simulink model "HydBrakeCU_ESP"  (Simulink 10.1)
settings: Solver=ode45  StartTime=0.0  StopTime=inf  RelTol=1e-3  EnableMultiTasking=on
PreLoadFcn:
  | HydBrakeCU_ESP_params
undefined symbols (not defined in the file): Area_Front, Area_Rear, ay_max_off, ay_max_on, ay_per_mu_max_off, ay_per_mu_max_on, Brake_ratio, brake_valve_ctrl_kP, cat1mode1_higher, cat1mode1_lower, cat1mode2_higher, cat1mode2_lower, cat1mode3_higher, cat1mode3_lower, cat2mode1_higher, cat2mode1_lower, cat2mode2_higher, cat2mode2_lower, cat2mode3_higher, cat2mode3_lower, delta_vel, diff_lock_fac, diff_lock_off, diff_lock_on, ESP_ctrl_kD, ESP_ctrl_kI, ESP_ctrl_kP, ESP_ctrl_restore_kI, ESP_min_throttle_fac, f_ax, f_slip, g, higherlimit_highvel, higherlimit_lowvel, highervel_fac, highervelocity_fac, InitialConditionForIntegrator, limit_acc, limit_selectlow, limit_starting, limit_vdiff, locktime_throttle, lowerlimit_highvel, lowerlimit_lowvel, lowervel_fac, lowervelocity_fac, min_throttle, MPS2KMPH, MSR_ctrl_kD, MSR_ctrl_kI, MSR_ctrl_kP, MSR_min_throttle_fac, PID_kP_sideslip, PID_kP_yawrate, RADpS2RpM, rBrake, RpM2RADpS, SH_SL_switch, sideslip_vel_corr, sidesplip_deviation_max ... (+33)
libraries: CarMaker4SL x136, simulink x49, simulink_extras x6
(part 5 of 6)

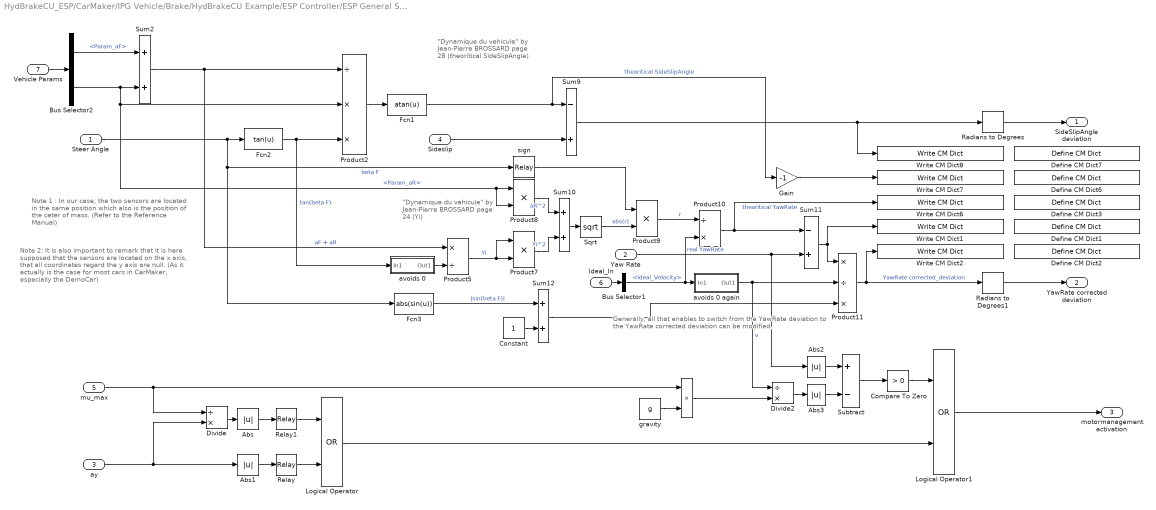
== system HydBrakeCU_ESP/CarMaker/IPG Vehicle/Brake/HydBrakeCU Example/ESP Controller/ESP General System/ESP/ECU/Instability detectors ==
  note: Note 1 :
      | In our case, the two sensors
      | are located in the same position
      | which also is the position of the ceter of mass.
      | (Refer to the Reference Manual)
  note: Note 2:
      | It is also important to remark that it is here
      | supposed that the sensors are located on the x axis,
      | that all coordinates regard the y axis are null.
      | (As it actually is the case for most cars in CarMaker,
      | especially the DemoCar)
  note: "Dynamique du vehicule"
      | by Jean-Pierre BROSSARD
      | page 28
      | (theoritical SideSlipAngle)
  note: Generally, all that enables to switch from the YawRate deviation
      | to the YawRate corrected deviation can be modified.
  note: "Dynamique du vehicule"
      | by Jean-Pierre BROSSARD
      | page 24
      | (Yi)
  Steer Angle : Inport
  Yaw Rate : Inport  Port=2
  ay : Inport  Port=3
  Sideslip : Inport  Port=4
  mu_max : Inport  Port=5
  Ideal_In : Inport  Port=6
  Vehicle Params : Inport  Port=7
  " " : Product  Inputs=**
  Abs{,1..3} (4 alike) : Abs
  Bus Selector1 : BusSelector  OutputSignals=Ideal_Velocity.Ideal_Velocity
  Bus Selector2 : BusSelector  OutputSignals=VehicleGeometry.Param_aF,VehicleGeometry.Param_aR
  Compare To Zero : simulink/Logic and Bit Operations/Compare To Zero  relop=>  OutDataTypeStr=uint8
  Constant : Constant
  Define CM Dict1 : CarMaker4SL/Define CM Dict  xname=ESP.YawRate_deviation  xunit=rad/s  xmono=off  xtype=Double4  xdvaplace=None  xnstates=0  xfirststate=0  xinitial=0
  Define CM Dict2 : CarMaker4SL/Define CM Dict  xname=ESP.YawRate_corrected_deviation  xunit=rad/m  xmono=off  xtype=Double4  xdvaplace=None  xnstates=0  xfirststate=0  xinitial=0
  Define CM Dict3 : CarMaker4SL/Define CM Dict  xname=ESP.YawRate_theoretical  xunit=rad/s  xmono=off  xtype=Double4  xdvaplace=None  xnstates=0  xfirststate=0  xinitial=0
  Define CM Dict6 : CarMaker4SL/Define CM Dict  xname=ESP.SideSlipeAngle_theoretical  xunit=rad  xmono=off  xtype=Double4  xdvaplace=None  xnstates=0  xfirststate=0  xinitial=0
  Define CM Dict7 : CarMaker4SL/Define CM Dict  xname=ESP.SideSlipAngle_deviation  xunit=rad  xmono=off  xtype=Double4  xdvaplace=None  xnstates=0  xfirststate=0  xinitial=0
  Divide : Product  Inputs=/*
  Divide2 : Product  Inputs=/*
  Fcn1 : Fcn  Expr=atan(u)
  Fcn2 : Fcn  Expr=tan(u)
  Fcn3 : Fcn  Expr=abs(sin(u))
  Gain : Gain  Gain=-1
  Logical Operator : Logic  Operator=OR  AllPortsSameDT=off  OutDataTypeStr=boolean
  Logical Operator1 : Logic  Operator=OR  AllPortsSameDT=off  OutDataTypeStr=boolean
  Product10 : Product  Inputs=/*  RndMeth=Zero
  Product11 : Product  Inputs=*/*  RndMeth=Zero
  Product2 : Product  Inputs=/**  RndMeth=Zero
  Product5 : Product  Inputs=*/  RndMeth=Zero
  Product7 : Product  RndMeth=Zero
  Product8 : Product  RndMeth=Zero
  Product9 : Product  RndMeth=Zero
  Radians to Degrees : simulink_extras/Transformations/Radians to Degrees
  Radians to Degrees1 : simulink_extras/Transformations/Radians to Degrees
  Relay : Relay  OnSwitchValue=ay_max_on  OffSwitchValue=ay_max_off
  Relay1 : Relay  OnSwitchValue=ay_per_mu_max_on  OffSwitchValue=ay_per_mu_max_off
  Sqrt : Math  Operator=sqrt  SignedPower=on  SaturateOnIntegerOverflow=on
  Subtract : Sum  Inputs=+-
  Sum10 : Sum  Inputs=2  InputSameDT=on  SaturateOnIntegerOverflow=on  OutDataTypeStr=Inherit: Same as first input
  Sum11 : Sum  Inputs=-+  InputSameDT=on  SaturateOnIntegerOverflow=on  OutDataTypeStr=Inherit: Same as first input
  Sum12 : Sum  InputSameDT=on  SaturateOnIntegerOverflow=on  OutDataTypeStr=Inherit: Same as first input
  Sum2 : Sum  Inputs=2  InputSameDT=on  SaturateOnIntegerOverflow=on  OutDataTypeStr=Inherit: Same as first input
  Sum9 : Sum  Inputs=-+  InputSameDT=on  SaturateOnIntegerOverflow=on  OutDataTypeStr=Inherit: Same as first input
  Write CM Dict1 : CarMaker4SL/Write CM Dict  xname=ESP.YawRate_deviation  xsync=off
  Write CM Dict2 : CarMaker4SL/Write CM Dict  xname=ESP.YawRate_corrected_deviation  xsync=off
  Write CM Dict6 : CarMaker4SL/Write CM Dict  xname=ESP.YawRate_theoretical  xsync=off
  Write CM Dict7 : CarMaker4SL/Write CM Dict  xname=ESP.SideSlipeAngle_theoretical  xsync=off
  Write CM Dict8 : CarMaker4SL/Write CM Dict  xname=ESP.SideSlipAngle_deviation  xsync=off
  avoids 0 : Subsystem
  avoids 0 again : Subsystem
  gravity : Constant  Value=g
  sign : Relay  OnSwitchValue=0  OffSwitchValue=0  OffOutputValue=-1
  SideSlipAngle deviation : Outport  VectorParamsAs1DForOutWhenUnconnected=off
  YawRate corrected deviation : Outport  Port=2  VectorParamsAs1DForOutWhenUnconnected=off
  motormanagement activation : Outport  Port=3  VectorParamsAs1DForOutWhenUnconnected=off
  wires:
  Steer Angle/1 -> Fcn2/1, sign/1, Fcn3/1  "beta F"
  Bus Selector2/1 -> Sum2/1  "<Param_aF>"
  Bus Selector2/2 -> Product8/1, Product8/2, Product2/2, Sum2/2  "<Param_aR>"
  Fcn2/1 -> avoids 0/1(In1), Product2/3  "tan(beta F)"
  Sum2/1 -> Product5/1, Product2/1  "aF + aR"
  Sum9/1 -> Radians to Degrees/1, Write CM Dict8/1
  Product2/1 -> Fcn1/1
  Fcn1/1 -> Sum9/1, Gain/1  "theoritical SideSlipAngle"
  Sideslip/1 -> Sum9/2
  Product5/1 -> Product7/2, Product7/1  "Yi"
  Product8/1 -> Sum10/1  "aR^2"
  Product7/1 -> Sum10/2  "Yi^2"
  Sum10/1 -> Sqrt/1
  Sqrt/1 -> Product9/2  "abs(r)"
  sign/1 -> Product9/1
  avoids 0/1(Out1) -> Product5/2
  Product9/1 -> Product10/1  "r"
  Product10/1 -> Sum11/1, Write CM Dict6/1  "theoritical YawRate"
  Yaw Rate/1 -> Sum11/2, Abs2/1  "real YawRate"
  Bus Selector1/1 -> Product10/2, avoids 0 again/1(In1)  "<Ideal_Velocity>"
  Constant/1 -> Sum12/2
  Product11/1 -> Radians to Degrees1/1, Write CM Dict2/1  "YawRate corrected_deviation"
  Sum11/1 -> Product11/1, Write CM Dict1/1
  Fcn3/1 -> Sum12/1  "|sin(beta F)|"
  avoids 0 again/1(Out1) -> Divide2/1, Product11/2  "v"
  Radians to Degrees/1 -> SideSlipAngle deviation/1
  Radians to Degrees1/1 -> YawRate corrected deviation/1
  Sum12/1 -> Product11/3
  Divide/1 -> Abs/1
  Abs/1 -> Relay1/1
  Abs1/1 -> Relay/1
  ay/1 -> Divide/2, Abs1/1
  mu_max/1 -> Divide/1, " "/1
  gravity/1 -> " "/2
  " "/1 -> Divide2/2
  Divide2/1 -> Abs3/1
  Abs2/1 -> Subtract/1
  Abs3/1 -> Subtract/2
  Subtract/1 -> Compare To Zero/1
  Logical Operator1/1 -> motormanagement activation/1
  Compare To Zero/1 -> Logical Operator1/1
  Logical Operator/1 -> Logical Operator1/2
  Relay1/1 -> Logical Operator/1
  Relay/1 -> Logical Operator/2
  Ideal_In/1 -> Bus Selector1/1
  Vehicle Params/1 -> Bus Selector2/1
  Gain/1 -> Write CM Dict7/1

== system HydBrakeCU_ESP/CarMaker/IPG Vehicle/Brake/HydBrakeCU Example/ESP Controller/ESP General System/ESP/ECU/Motor management strategy ==
  activation DK : Inport
  Throttle_position : Inport  Port=2
  ax : Inport  Port=3
  Abs1 : Abs
  Compare To Zero : simulink/Logic and Bit Operations/Compare To Zero  relop===  OutDataTypeStr=uint8
  Constant : Constant  Value=ESP_min_throttle_fac
  Data Type Conversion2 : DataTypeConversion
  PID-Controller : Subsystem
  Product : Product  RndMeth=Zero
  Saturation Dynamic : simulink/Discontinuities/Saturation Dynamic  OutMin=[]  OutMax=[]  OutDataTypeStr=Inherit: Same as second input  OutDataType=sfix(16)  OutScaling=2^-10  DoSatur=off
  Switch1 : Switch  Criteria=u2 > Threshold
  Switch3 : Switch  Criteria=u2 > Threshold
  restoration to driver : Subsystem
  vquer_VA1 : Gain
  Gas_out : Outport  VectorParamsAs1DForOutWhenUnconnected=off
  wires:
  Compare To Zero/1 -> Data Type Conversion2/1
  Data Type Conversion2/1 -> PID-Controller/2(RESET)
  Throttle_position/1 -> Switch3/3, Product/1, vquer_VA1/1
  vquer_VA1/1 -> Saturation Dynamic/1
  Product/1 -> Saturation Dynamic/3
  activation DK/1 -> Compare To Zero/1, Switch3/2, restoration to driver/2(activation on)
  PID-Controller/1(y) -> Saturation Dynamic/2
  Saturation Dynamic/1 -> Switch3/1, restoration to driver/1(controller in)
  Switch3/1 -> Switch1/3, restoration to driver/3(driver in)
  Switch1/1 -> Gas_out/1
  restoration to driver/1(Control Gas) -> Switch1/1
  ax/1 -> Abs1/1
  Abs1/1 -> PID-Controller/1(u)
  restoration to driver/2(restoration) -> Switch1/2
  Constant/1 -> Product/2

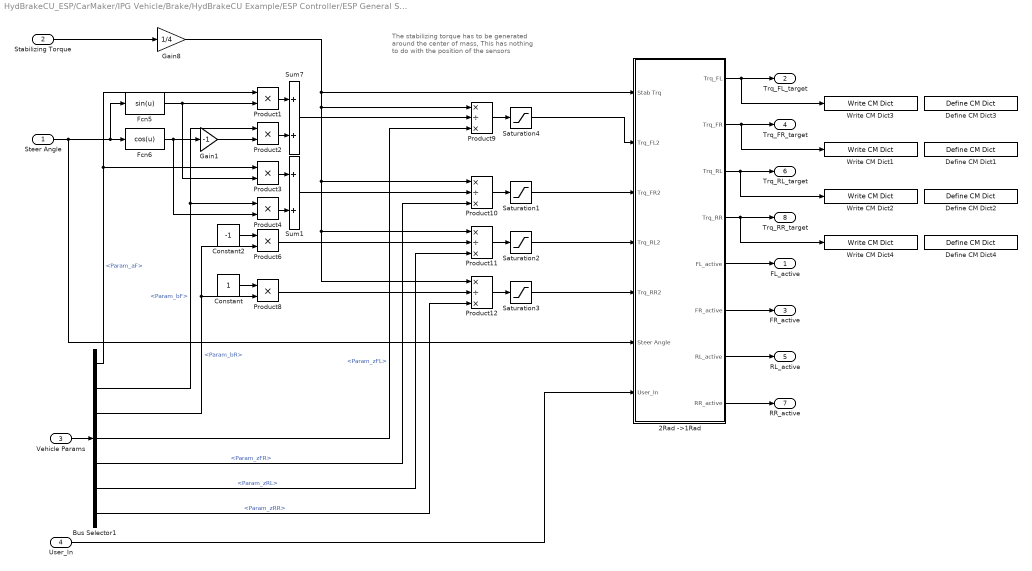
== system HydBrakeCU_ESP/CarMaker/IPG Vehicle/Brake/HydBrakeCU Example/ESP Controller/ESP General System/ESP/ECU/brake distribution strategy ==
  note: The stabilizing torque has to be generated
      | around the center of mass,
      | This has nothing to do with
      | the position of the sensors
  Steer Angle : Inport
  Stabilizing Torque : Inport  Port=2
  Vehicle Params : Inport  Port=3
  User_In : Inport  Port=4
  2Rad ->1Rad : Subsystem
  Bus Selector1 : BusSelector  OutputSignals=VehicleGeometry.Param_aF,VehicleGeometry.Param_bF,VehicleGeometry.Param_bR,CarrierGeometry.Param_zFL,CarrierGeometry.Param_zFR,CarrierGeometry.Param_zRL,CarrierGeometry.Param_zRR
  Constant : Constant
  Constant2 : Constant  Value=-1
  Define CM Dict1 : CarMaker4SL/Define CM Dict  xname=ESP.ESP_corr_Trq_FR  xunit=Nm  xmono=off  xtype=Double4  xdvaplace=None  xnstates=0  xfirststate=0  xinitial=0
  Define CM Dict2 : CarMaker4SL/Define CM Dict  xname=ESP.ESP_corr_Trq_RL  xunit=Nm  xmono=off  xtype=Double4  xdvaplace=None  xnstates=0  xfirststate=0  xinitial=0
  Define CM Dict3 : CarMaker4SL/Define CM Dict  xname=ESP.ESP_corr_Trq_FL  xunit=Nm  xmono=off  xtype=Double4  xdvaplace=None  xnstates=0  xfirststate=0  xinitial=0
  Define CM Dict4 : CarMaker4SL/Define CM Dict  xname=ESP.ESP_corr_Trq_RR  xunit=Nm  xmono=off  xtype=Double4  xdvaplace=None  xnstates=0  xfirststate=0  xinitial=0
  Fcn5 : Fcn  Expr=sin(u)
  Fcn6 : Fcn  Expr=cos(u)
  Gain1 : Gain  Gain=-1
  Gain8 : Gain  Gain=1/4
  Product{1..4,6,8} (6 alike) : Product  RndMeth=Zero
  Product{9..12} (4 alike) : Product  Inputs=*/*  RndMeth=Zero
  Saturation{1..4} (4 alike) : Saturate  UpperLimit=3000  LowerLimit=-3000
  Sum1 : Sum  Inputs=2  InputSameDT=on  SaturateOnIntegerOverflow=on  OutDataTypeStr=Inherit: Same as first input
  Sum7 : Sum  Inputs=2  InputSameDT=on  SaturateOnIntegerOverflow=on  OutDataTypeStr=Inherit: Same as first input
  Write CM Dict1 : CarMaker4SL/Write CM Dict  xname=ESP.ESP_corr_Trq_FR  xsync=off
  Write CM Dict2 : CarMaker4SL/Write CM Dict  xname=ESP.ESP_corr_Trq_RL  xsync=off
  Write CM Dict3 : CarMaker4SL/Write CM Dict  xname=ESP.ESP_corr_Trq_FL  xsync=off
  Write CM Dict4 : CarMaker4SL/Write CM Dict  xname=ESP.ESP_corr_Trq_RR  xsync=off
  FL_active : Outport  VectorParamsAs1DForOutWhenUnconnected=off
  Trq_FL_target : Outport  Port=2  VectorParamsAs1DForOutWhenUnconnected=off
  FR_active : Outport  Port=3  VectorParamsAs1DForOutWhenUnconnected=off
  Trq_FR_target : Outport  Port=4  VectorParamsAs1DForOutWhenUnconnected=off
  RL_active : Outport  Port=5  VectorParamsAs1DForOutWhenUnconnected=off
  Trq_RL_target : Outport  Port=6  VectorParamsAs1DForOutWhenUnconnected=off
  RR_active : Outport  Port=7  VectorParamsAs1DForOutWhenUnconnected=off
  Trq_RR_target : Outport  Port=8  VectorParamsAs1DForOutWhenUnconnected=off
  wires:
  Steer Angle/1 -> Fcn5/1, Fcn6/1, 2Rad ->1Rad/6(Steer Angle)
  Fcn5/1 -> Product1/2, Product3/2
  Fcn6/1 -> Product4/2, Gain1/1
  Gain1/1 -> Product2/2
  Product1/1 -> Sum7/1
  Product2/1 -> Sum7/2
  Product3/1 -> Sum1/1
  Product4/1 -> Sum1/2
  Product6/1 -> Product11/2
  Product8/1 -> Product12/2
  Sum1/1 -> Product10/2
  Sum7/1 -> Product9/2
  Product9/1 -> Saturation4/1
  Saturation4/1 -> 2Rad ->1Rad/2(Trq_FL2)
  Saturation1/1 -> 2Rad ->1Rad/3(Trq_FR2)
  Saturation3/1 -> 2Rad ->1Rad/5(Trq_RR2)
  Saturation2/1 -> 2Rad ->1Rad/4(Trq_RL2)
  Stabilizing Torque/1 -> Gain8/1
  Gain8/1 -> Product12/1, Product11/1, Product10/1, Product9/1, 2Rad ->1Rad/1(Stab Trq)
  Product10/1 -> Saturation1/1
  Product12/1 -> Saturation3/1
  Product11/1 -> Saturation2/1
  Bus Selector1/3 -> Product6/2, Product8/2  "<Param_bR>"
  Bus Selector1/2 -> Product4/1, Product2/1  "<Param_bF>"
  2Rad ->1Rad/2(Trq_FR) -> Write CM Dict1/1, Trq_FR_target/1
  2Rad ->1Rad/3(Trq_RL) -> Write CM Dict2/1, Trq_RL_target/1
  2Rad ->1Rad/4(Trq_RR) -> Trq_RR_target/1, Write CM Dict4/1
  2Rad ->1Rad/5(FL_active) -> FL_active/1
  2Rad ->1Rad/6(FR_active) -> FR_active/1
  2Rad ->1Rad/7(RL_active) -> RL_active/1
  2Rad ->1Rad/8(RR_active) -> RR_active/1
  Vehicle Params/1 -> Bus Selector1/1
  Bus Selector1/1 -> Product3/1, Product1/1  "<Param_aF>"
  Constant2/1 -> Product6/1
  Constant/1 -> Product8/1
  Bus Selector1/4 -> Product9/3  "<Param_zFL>"
  Bus Selector1/5 -> Product10/3  "<Param_zFR>"
  Bus Selector1/6 -> Product11/3  "<Param_zRL>"
  Bus Selector1/7 -> Product12/3  "<Param_zRR>"
  User_In/1 -> 2Rad ->1Rad/7(User_In)
  2Rad ->1Rad/1(Trq_FL) -> Write CM Dict3/1, Trq_FL_target/1

== system HydBrakeCU_ESP/CarMaker/IPG Vehicle/Brake/HydBrakeCU Example/ESP Controller/ESP General System/ESP/helpsignals estimator/SideSlip estimator ==
  lenkwinkel : Inport
  CarMaker_In : Inport  Port=2
  Bus Selector1 : BusSelector  OutputSignals=Ideal_Velocity.Ideal_Velocity_y,Ideal_Velocity.Ideal_Velocity_x
  Constant1 : Constant  Value=0
  Divide6 : Product  Inputs=*/
  Switch : Switch  Threshold=1
  Terminator : Terminator
  Trigonometric Function2 : Trigonometry  Operator=atan
  SideSlipAngle_estimated : Outport  VectorParamsAs1DForOutWhenUnconnected=off
  wires:
  Bus Selector1/2 -> Divide6/2, Switch/2  "<Ideal_Velocity_x>"
  Divide6/1 -> Trigonometric Function2/1
  Trigonometric Function2/1 -> Switch/1
  Constant1/1 -> Switch/3
  Switch/1 -> SideSlipAngle_estimated/1
  lenkwinkel/1 -> Terminator/1
  CarMaker_In/1 -> Bus Selector1/1
  Bus Selector1/1 -> Divide6/1  "<Ideal_Velocity_y>"

== system HydBrakeCU_ESP/CarMaker/IPG Vehicle/Brake/HydBrakeCU Example/ESP Controller/ESP General System/ESP/helpsignals estimator/mue estimator ==
  CarMaker_In : Inport
  Vehicle Params : Inport  Port=2
  Bus Selector1 : BusSelector  OutputSignals=Idea_Trq2W.Ideal_Trq2WRL,Ideal_Fz.Ideal_FzRL,Ideal_Slip.Ideal_SlipRL,Ideal_Velocity.Ideal_Velocity_x,Ideal_YawRate
  Bus Selector2 : BusSelector  OutputSignals=TireRadius.Param_RadiusRL,TireRadius.Param_RadiusRR
  Bus Selector3 : BusSelector  OutputSignals=Idea_Trq2W.Ideal_Trq2WRR,Ideal_Fz.Ideal_FzRR,Ideal_Slip.Ideal_SlipRR,Ideal_Velocity.Ideal_Velocity_x,Ideal_YawRate
  MinMax : MinMax  Inputs=2
  estimator_RL : Subsystem
  estimator_RR : Subsystem
  mue_estimated : Outport  VectorParamsAs1DForOutWhenUnconnected=off
  wires:
  MinMax/1 -> mue_estimated/1
  estimator_RL/1(mue_est_RL) -> MinMax/1
  estimator_RR/1(mue_est_RR) -> MinMax/2
  CarMaker_In/1 -> Bus Selector3/1, Bus Selector1/1
  Vehicle Params/1 -> Bus Selector2/1
  Bus Selector2/1 -> estimator_RL/6(Radius_RL)  "<Param_RadiusRL>"
  Bus Selector2/2 -> estimator_RR/6(Radius_RR)  "<Param_RadiusRR>"
  Bus Selector1/3 -> estimator_RL/3(LongSlip_RL)  "<Ideal_SlipRL>"
  Bus Selector1/4 -> estimator_RL/4(Car_vx)  "<Ideal_Velocity_x>"
  Bus Selector1/2 -> estimator_RL/2(Fz_RL)  "<Ideal_FzRL>"
  Bus Selector1/5 -> estimator_RL/5(YawRate)  "<Ideal_YawRate>"
  Bus Selector1/1 -> estimator_RL/1(Trq2W_RL)  "<Ideal_Trq2WRL>"
  Bus Selector3/1 -> estimator_RR/1(Trq2W_RR)  "<Ideal_Trq2WRR>"
  Bus Selector3/2 -> estimator_RR/2(Fz_RR)  "<Ideal_FzRR>"
  Bus Selector3/3 -> estimator_RR/3(LongSlip_RR)  "<Ideal_SlipRR>"
  Bus Selector3/4 -> estimator_RR/4(Car_vx)  "<Ideal_Velocity_x>"
  Bus Selector3/5 -> estimator_RR/5(YawRate)  "<Ideal_YawRate>"

== system HydBrakeCU_ESP/CarMaker/IPG Vehicle/Brake/HydBrakeCU Example/ESP Controller/ESP General System/ABS/ABS ECU/ABS_ValveCtrl_FL/Duty ==
  Constant1 : Constant  Value=1/t_Sensor
  Integrator : Integrator  ExternalReset=either
  Pulse Generator : DiscretePulseGenerator  PulseType=Time based  Period=t_Sensor*2  PulseWidth=50
  SZ : Outport  VectorParamsAs1DForOutWhenUnconnected=off
  wires:
  Pulse Generator/1 -> Integrator/2
  Constant1/1 -> Integrator/1
  Integrator/1 -> SZ/1

== system HydBrakeCU_ESP/CarMaker/IPG Vehicle/Brake/HydBrakeCU Example/ESP Controller/ESP General System/ABS/ABS ECU/ABS_ValveCtrl_FR/Duty ==
  Constant1 : Constant  Value=1/t_Sensor
  Integrator : Integrator  ExternalReset=either
  Pulse Generator : DiscretePulseGenerator  PulseType=Time based  Period=t_Sensor*2  PulseWidth=50
  SZ : Outport  VectorParamsAs1DForOutWhenUnconnected=off
  wires:
  Integrator/1 -> SZ/1
  Pulse Generator/1 -> Integrator/2
  Constant1/1 -> Integrator/1

== system HydBrakeCU_ESP/CarMaker/IPG Vehicle/Brake/HydBrakeCU Example/ESP Controller/ESP General System/ABS/ABS ECU/select_low/ABS_ValveCtrl_rear ==
  note: Valve Control:
      | Valves are open for a predefined time window.
      | The driving time depends on a trigger criterion (LUT).
      | The treshold change for the valve driving time is
      | continously modified by a repeating sequence.
  note: EITHER ABS is switched on and  S_K is put through
      |  when S_K is becomming bigger the s_{ku}
      | OR output is 0 when S_K is smaller than {sku}_{off}
  Sk : Inport
  Constant : Constant
  Duty : Subsystem
  Look-Up Table1 : Lookup  InputValues=Valve_LUTin_HA  Table=ValveIn_LUTout_HA  LookUpMeth=Interpolation-Use End Values  SaturateOnIntegerOverflow=on
  Look-Up Table2 : Lookup  InputValues=Valve_LUTin_HA  Table=ValveOut_LUTout_HA  LookUpMeth=Interpolation-Use End Values  SaturateOnIntegerOverflow=on
  Product : Product  SaturateOnIntegerOverflow=on  OutDataTypeStr=Inherit: Same as first input
  Rate Transition{1..4} (4 alike) : RateTransition
  Relational Operator : RelationalOperator  Operator=<  SampleTime=0.001  RndMeth=Nearest
  Relational Operator1 : RelationalOperator  Operator=<  SampleTime=0.001  RndMeth=Nearest
  Relay : Relay  OnSwitchValue=sku_HA  OffSwitchValue=sku_off_HA
  Sum1 : Sum  Inputs=--+  SaturateOnIntegerOverflow=on
  Zero-Order Hold : ZeroOrderHold  SampleTime=t_Sensor
  Brake.Valve.In : Outport  VectorParamsAs1DForOutWhenUnconnected=off
  Brake.Valve.Out : Outport  Port=2  VectorParamsAs1DForOutWhenUnconnected=off
  Brake.ABS.status : Outport  Port=3  VectorParamsAs1DForOutWhenUnconnected=off
  Brake.ABS.on/off : Outport  Port=4  VectorParamsAs1DForOutWhenUnconnected=off
  wires:
  Sk/1 -> Zero-Order Hold/1
  Product/1 -> Look-Up Table1/1, Look-Up Table2/1
  Relay/1 -> Rate Transition4/1, Product/2
  Zero-Order Hold/1 -> Product/1, Relay/1
  Look-Up Table2/1 -> Rate Transition3/1
  Look-Up Table1/1 -> Rate Transition1/1
  Duty/1(SZ) -> Rate Transition2/1
  Sum1/1 -> Brake.ABS.status/1
  Constant/1 -> Sum1/3
  Relational Operator1/1 -> Sum1/2, Brake.Valve.Out/1
  Relational Operator/1 -> Sum1/1, Brake.Valve.In/1
  Rate Transition2/1 -> Relational Operator1/1, Relational Operator/1
  Rate Transition1/1 -> Relational Operator/2
  Rate Transition3/1 -> Relational Operator1/2
  Rate Transition4/1 -> Brake.ABS.on/off/1

== system HydBrakeCU_ESP/CarMaker/IPG Vehicle/Brake/HydBrakeCU Example/ESP Controller/ESP General System/ASR/BMR ECU/BMR Controller/If Action Subsystem10 ==
  Action Port : ActionPort  ActionPortLabel=else { }
  Constant3 : Constant  Value=ValveIn_abbau
  Constant4 : Constant  Value=ValveOut_abbau
  Out1 : Outport  InitialOutput=[ValveIn_abbau]  VectorParamsAs1DForOutWhenUnconnected=off
  Out2 : Outport  Port=2  InitialOutput=[ValveOut_abbau]  VectorParamsAs1DForOutWhenUnconnected=off
  wires:
  Constant3/1 -> Out1/1
  Constant4/1 -> Out2/1

== system HydBrakeCU_ESP/CarMaker/IPG Vehicle/Brake/HydBrakeCU Example/ESP Controller/ESP General System/ASR/BMR ECU/BMR Controller/If Action Subsystem11 ==
  Action Port : ActionPort  ActionPortLabel=else { }
  Constant3 : Constant  Value=ValveIn_abbau
  Constant4 : Constant  Value=ValveOut_abbau
  Out1 : Outport  InitialOutput=[ValveIn_abbau]  VectorParamsAs1DForOutWhenUnconnected=off
  Out2 : Outport  Port=2  InitialOutput=[ValveOut_abbau]  VectorParamsAs1DForOutWhenUnconnected=off
  wires:
  Constant3/1 -> Out1/1
  Constant4/1 -> Out2/1

== system HydBrakeCU_ESP/CarMaker/IPG Vehicle/Brake/HydBrakeCU Example/ESP Controller/ESP General System/ASR/BMR ECU/BMR Controller/If Action Subsystem12 ==
  Action Port : ActionPort  ActionPortLabel=if { }
  Constant2 : Constant  Value=ValveIn_aufbau_long
  Constant3 : Constant  Value=ValveOut_aufbau_long
  Out1 : Outport  InitialOutput=[ValveIn_aufbau_long]  VectorParamsAs1DForOutWhenUnconnected=off
  Out2 : Outport  Port=2  InitialOutput=[ValveOut_aufbau_long]  VectorParamsAs1DForOutWhenUnconnected=off
  wires:
  Constant3/1 -> Out2/1
  Constant2/1 -> Out1/1

== system HydBrakeCU_ESP/CarMaker/IPG Vehicle/Brake/HydBrakeCU Example/ESP Controller/ESP General System/ASR/BMR ECU/BMR Controller/If Action Subsystem13 ==
  Action Port : ActionPort  ActionPortLabel=elseif { }
  Constant2 : Constant  Value=ValveIn_aufbau_short
  Constant3 : Constant  Value=ValveOut_aufbau_short
  Out1 : Outport  InitialOutput=[ValveIn_aufbau_short]  VectorParamsAs1DForOutWhenUnconnected=off
  Out2 : Outport  Port=2  InitialOutput=[ValveOut_aufbau_short]  VectorParamsAs1DForOutWhenUnconnected=off
  wires:
  Constant2/1 -> Out1/1
  Constant3/1 -> Out2/1

== system HydBrakeCU_ESP/CarMaker/IPG Vehicle/Brake/HydBrakeCU Example/ESP Controller/ESP General System/ASR/BMR ECU/BMR Controller/If Action Subsystem8 ==
  Action Port : ActionPort  ActionPortLabel=if { }
  Constant2 : Constant  Value=ValveIn_aufbau_long
  Constant3 : Constant  Value=ValveOut_aufbau_long
  Out1 : Outport  InitialOutput=[ValveIn_aufbau_long]  VectorParamsAs1DForOutWhenUnconnected=off
  Out2 : Outport  Port=2  InitialOutput=[ValveOut_aufbau_long]  VectorParamsAs1DForOutWhenUnconnected=off
  wires:
  Constant2/1 -> Out1/1
  Constant3/1 -> Out2/1

== system HydBrakeCU_ESP/CarMaker/IPG Vehicle/Brake/HydBrakeCU Example/ESP Controller/ESP General System/ASR/BMR ECU/BMR Controller/If Action Subsystem9 ==
  Action Port : ActionPort  ActionPortLabel=elseif { }
  Constant2 : Constant  Value=ValveIn_aufbau_short
  Constant3 : Constant  Value=ValveOut_aufbau_short
  Out1 : Outport  InitialOutput=[ValveIn_aufbau_short]  VectorParamsAs1DForOutWhenUnconnected=off
  Out2 : Outport  Port=2  InitialOutput=[ValveOut_aufbau_short]  VectorParamsAs1DForOutWhenUnconnected=off
  wires:
  Constant2/1 -> Out1/1
  Constant3/1 -> Out2/1

== system HydBrakeCU_ESP/CarMaker/IPG Vehicle/Brake/HydBrakeCU Example/ESP Controller/ESP General System/ASR/BMR ECU/BMR Controller/Pulsing ==
  Constant1 : Constant  Value=1/t_Sensor
  Integrator : Integrator  ExternalReset=either
  Pulse Generator : DiscretePulseGenerator  PulseType=Time based  Period=t_Sensor*2  PulseWidth=50
  SZ : Outport  VectorParamsAs1DForOutWhenUnconnected=off
  wires:
  Pulse Generator/1 -> Integrator/2
  Constant1/1 -> Integrator/1
  Integrator/1 -> SZ/1

== system HydBrakeCU_ESP/CarMaker/IPG Vehicle/Brake/HydBrakeCU Example/ESP Controller/ESP General System/ASR/BMR ECU/BMR Controller/Pulsing1 ==
  Constant1 : Constant  Value=1/t_Sensor
  Integrator : Integrator  ExternalReset=either
  Pulse Generator : DiscretePulseGenerator  PulseType=Time based  Period=t_Sensor*2  PulseWidth=50
  SZ : Outport  VectorParamsAs1DForOutWhenUnconnected=off
  wires:
  Integrator/1 -> SZ/1
  Constant1/1 -> Integrator/1
  Pulse Generator/1 -> Integrator/2

== system HydBrakeCU_ESP/CarMaker/IPG Vehicle/Brake/HydBrakeCU Example/ESP Controller/ESP General System/ASR/BMR ECU/BMR Controller/Signal Mapping ==
  User_In : Inport
  Valve_In_DrivenL : Inport  Port=2
  Valve_Out_DrivenL : Inport  Port=3
  Valve_In_DrivenR : Inport  Port=4
  Valve_Out_DrivenR : Inport  Port=5
  Valve_In_Undriven : Inport  Port=6
  Valve_Out_Undriven : Inport  Port=7
  Valves_Drivenaxle : Inport  Port=8
  Valves_Undrivenaxle : Inport  Port=9
  Bus Selector2 : BusSelector  OutputSignals=User_Drive
  Demux2 : Demux  Outputs=13
  Mux1 : Mux  Inputs=13
  Mux2 : Mux  Inputs=13
  Mux3 : Mux  Inputs=13
  Switch2 : Switch  Criteria=u2 > Threshold  Threshold=1.5
  Switch3 : Switch  Criteria=u2 > Threshold  Threshold=2.5
  Brake Valve_In_FL : Outport  VectorParamsAs1DForOutWhenUnconnected=off
  Brake Valve_In_FR : Outport  Port=2  VectorParamsAs1DForOutWhenUnconnected=off
  Brake Valve_In_RL : Outport  Port=3  VectorParamsAs1DForOutWhenUnconnected=off
  Brake Valve_In_RR : Outport  Port=4  VectorParamsAs1DForOutWhenUnconnected=off
  Brake Valve_Out_FL : Outport  Port=5  VectorParamsAs1DForOutWhenUnconnected=off
  Brake Valve_Out_FR : Outport  Port=6  VectorParamsAs1DForOutWhenUnconnected=off
  Brake Valve_Out_RL : Outport  Port=7  VectorParamsAs1DForOutWhenUnconnected=off
  Brake Valve_Out_RR : Outport  Port=8  VectorParamsAs1DForOutWhenUnconnected=off
  Valve_PV_0 : Outport  Port=9  VectorParamsAs1DForOutWhenUnconnected=off
  Valve_PV_1 : Outport  Port=10  VectorParamsAs1DForOutWhenUnconnected=off
  Valve_SV_0 : Outport  Port=11  VectorParamsAs1DForOutWhenUnconnected=off
  Valve_SV_1 : Outport  Port=12  VectorParamsAs1DForOutWhenUnconnected=off
  Pump Ctrl : Outport  Port=13  VectorParamsAs1DForOutWhenUnconnected=off
  wires:
  Valve_In_Undriven/1 -> Mux2/1, Mux2/2, Mux1/5, Mux1/6
  Valve_Out_Undriven/1 -> Mux2/3, Mux2/4, Mux1/7, Mux1/8
  Valve_In_DrivenR/1 -> Mux2/7, Mux1/3, Mux3/7, Mux3/3
  Valve_In_DrivenL/1 -> Mux3/5, Mux3/1, Mux2/5, Mux1/1
  Valves_Undrivenaxle/1 -> Mux1/12, Mux1/11, Mux2/9, Mux2/10
  Valves_Drivenaxle/1 -> Mux1/9, Mux2/11, Mux2/12, Mux2/13, Mux1/10, Mux1/13, Mux3/10, Mux3/9, Mux3/11, Mux3/12, Mux3/13
  Valve_Out_DrivenL/1 -> Mux3/6, Mux3/2, Mux1/2, Mux2/6
  Valve_Out_DrivenR/1 -> Mux2/8, Mux3/4, Mux3/8, Mux1/4
  User_In/1 -> Bus Selector2/1
  Bus Selector2/1 -> Switch2/2, Switch3/2  "<User_Drive>"
  Switch2/1 -> Switch3/3
  Switch3/1 -> Demux2/1
  Mux1/1 -> Switch2/3
  Mux2/1 -> Switch2/1
  Demux2/1 -> Brake Valve_In_FL/1
  Demux2/2 -> Brake Valve_Out_FL/1
  Demux2/3 -> Brake Valve_In_FR/1
  Demux2/4 -> Brake Valve_Out_FR/1
  Demux2/5 -> Brake Valve_In_RL/1
  Demux2/6 -> Brake Valve_In_RR/1
  Demux2/7 -> Brake Valve_Out_RL/1
  Demux2/8 -> Brake Valve_Out_RR/1
  Demux2/9 -> Valve_PV_0/1
  Demux2/10 -> Valve_SV_0/1
  Demux2/11 -> Valve_PV_1/1
  Demux2/12 -> Valve_SV_1/1
  Demux2/13 -> Pump Ctrl/1
  Mux3/1 -> Switch3/1

== system HydBrakeCU_ESP/CarMaker/IPG Vehicle/Brake/HydBrakeCU Example/ESP Controller/ESP General System/ASR/BMR ECU/BMR logic/If Action Subsystem6 ==
  Action Port : ActionPort  ActionPortLabel=case: { }
  Constant : Constant  Value=higherlimit_lowvel
  Constant1 : Constant  Value=lowerlimit_lowvel
  Mux1 : Mux  Inputs=2
  1 : Outport  InitialOutput=[higherlimit_lowvel, lowerlimit_lowvel]  VectorParamsAs1DForOutWhenUnconnected=off
  wires:
  Mux1/1 -> 1/1
  Constant1/1 -> Mux1/2
  Constant/1 -> Mux1/1

== system HydBrakeCU_ESP/CarMaker/IPG Vehicle/Brake/HydBrakeCU Example/ESP Controller/ESP General System/ASR/BMR ECU/BMR logic/If Action Subsystem7 ==
  Action Port : ActionPort  ActionPortLabel=case: { }
  Constant : Constant  Value=higherlimit_highvel
  Constant1 : Constant  Value=lowerlimit_highvel
  Mux1 : Mux  Inputs=2
  2 : Outport  InitialOutput=[higherlimit_highvel, lowerlimit_highvel]  VectorParamsAs1DForOutWhenUnconnected=off
  wires:
  Constant/1 -> Mux1/1
  Constant1/1 -> Mux1/2
  Mux1/1 -> 2/1

== system HydBrakeCU_ESP/CarMaker/IPG Vehicle/Brake/HydBrakeCU Example/ESP Controller/ESP General System/ASR/BMR ECU/BMR logic/operating category ==
  note: Criteria of operating categories (Betriebsarten): Burckhardt: Fahrwerktechnik p.186f.
  v_RL : Inport
  v_RR : Inport  Port=2
  " " : RelationalOperator  Operator=>  OutDataTypeStr=boolean  RndMeth=Nearest
  "  " : Gain  Gain=0.5
  " 1" : RelationalOperator  Operator=<=  OutDataTypeStr=boolean  RndMeth=Nearest
  Add : Sum
  Add1 : Sum
  Constant1 : Constant  Value=delta_vel
  Constant2 : Constant  Value=delta_vel
  Data Type Conversion : DataTypeConversion
  Data Type Conversion1 : DataTypeConversion
  Data Type Conversion2 : DataTypeConversion
  vquer_HA2 : Gain
  vquer_HA3 : Gain  Gain=2
  operating category : Outport  VectorParamsAs1DForOutWhenUnconnected=off
  wires:
  " 1"/1 -> Data Type Conversion1/1
  " "/1 -> Data Type Conversion2/1
  Data Type Conversion/1 -> operating category/1
  Add1/1 -> Data Type Conversion/1
  vquer_HA3/1 -> Add1/2
  vquer_HA2/1 -> Add1/1
  "  "/1 -> " 1"/1, " "/1
  v_RL/1 -> Add/1
  Add/1 -> "  "/1
  v_RR/1 -> Add/2
  Constant2/1 -> " "/2
  Constant1/1 -> " 1"/2
  Data Type Conversion1/1 -> vquer_HA2/1
  Data Type Conversion2/1 -> vquer_HA3/1

== system HydBrakeCU_ESP/CarMaker/IPG Vehicle/Brake/HydBrakeCU Example/ESP Controller/ESP General System/ASR/MSR ECU/MSR logic/If Action Subsystem ==
  Action Port : ActionPort  ActionPortLabel=case: { }
  Constant : Constant  Value=cat1mode1_higher
  Constant1 : Constant  Value=cat1mode1_lower
  Mux1 : Mux  Inputs=2
  1.1 : Outport  InitialOutput=[cat1mode1_higher, cat1mode1_lower]  VectorParamsAs1DForOutWhenUnconnected=off
  wires:
  Constant/1 -> Mux1/1
  Constant1/1 -> Mux1/2
  Mux1/1 -> 1.1/1

== system HydBrakeCU_ESP/CarMaker/IPG Vehicle/Brake/HydBrakeCU Example/ESP Controller/ESP General System/ASR/MSR ECU/MSR logic/If Action Subsystem1 ==
  Action Port : ActionPort  ActionPortLabel=case: { }
  Constant : Constant  Value=cat1mode2_higher
  Constant1 : Constant  Value=cat1mode2_lower
  Mux1 : Mux  Inputs=2
  1.2 : Outport  InitialOutput=[cat1mode2_higher, cat1mode2_lower]  VectorParamsAs1DForOutWhenUnconnected=off
  wires:
  Mux1/1 -> 1.2/1
  Constant1/1 -> Mux1/2
  Constant/1 -> Mux1/1

== system HydBrakeCU_ESP/CarMaker/IPG Vehicle/Brake/HydBrakeCU Example/ESP Controller/ESP General System/ASR/MSR ECU/MSR logic/If Action Subsystem2 ==
  Action Port : ActionPort  ActionPortLabel=case: { }
  Constant2 : Constant  Value=cat1mode3_higher
  Constant3 : Constant  Value=cat1mode3_lower
  Mux1 : Mux  Inputs=2
  1.3 : Outport  InitialOutput=[cat1mode3_higher, cat1mode3_lower]  VectorParamsAs1DForOutWhenUnconnected=off
  wires:
  Mux1/1 -> 1.3/1
  Constant2/1 -> Mux1/1
  Constant3/1 -> Mux1/2

== system HydBrakeCU_ESP/CarMaker/IPG Vehicle/Brake/HydBrakeCU Example/ESP Controller/ESP General System/ASR/MSR ECU/MSR logic/If Action Subsystem3 ==
  Action Port : ActionPort  ActionPortLabel=case: { }
  Constant2 : Constant  Value=cat2mode1_higher
  Constant3 : Constant  Value=cat2mode1_lower
  Mux1 : Mux  Inputs=2
  2.1 : Outport  InitialOutput=[cat2mode1_higher, cat2mode1_lower]  VectorParamsAs1DForOutWhenUnconnected=off
  wires:
  Mux1/1 -> 2.1/1
  Constant3/1 -> Mux1/2
  Constant2/1 -> Mux1/1

== system HydBrakeCU_ESP/CarMaker/IPG Vehicle/Brake/HydBrakeCU Example/ESP Controller/ESP General System/ASR/MSR ECU/MSR logic/If Action Subsystem4 ==
  Action Port : ActionPort  ActionPortLabel=case: { }
  Constant2 : Constant  Value=cat2mode2_higher
  Constant3 : Constant  Value=cat2mode2_lower
  Mux1 : Mux  Inputs=2
  2.2 : Outport  InitialOutput=[cat2mode2_higher, cat2mode2_lower]  VectorParamsAs1DForOutWhenUnconnected=off
  wires:
  Mux1/1 -> 2.2/1
  Constant2/1 -> Mux1/1
  Constant3/1 -> Mux1/2

== system HydBrakeCU_ESP/CarMaker/IPG Vehicle/Brake/HydBrakeCU Example/ESP Controller/ESP General System/ASR/MSR ECU/MSR logic/If Action Subsystem5 ==
  Action Port : ActionPort  ActionPortLabel=case: { }
  Constant2 : Constant  Value=cat2mode3_higher
  Constant3 : Constant  Value=cat2mode3_lower
  Mux1 : Mux  Inputs=2
  2.3 : Outport  InitialOutput=[cat2mode3_higher, cat2mode3_lower]  VectorParamsAs1DForOutWhenUnconnected=off
  wires:
  Mux1/1 -> 2.3/1
  Constant2/1 -> Mux1/1
  Constant3/1 -> Mux1/2

== system HydBrakeCU_ESP/CarMaker/IPG Vehicle/Brake/HydBrakeCU Example/ESP Controller/ESP General System/ASR/MSR ECU/MSR logic/operating category ==
  note: Criteria of operating categories (Betriebsarten) - Burckhardt: Fahrwerktechnik p.174f.
  v_drivenL : Inport
  v_drivenR : Inport  Port=2
  v_undrivenL : Inport  Port=3
  v_undrivenR : Inport  Port=4
  " " : RelationalOperator  OutDataTypeStr=boolean  RndMeth=Nearest
  " 1" : RelationalOperator  Operator=<=  OutDataTypeStr=boolean  RndMeth=Nearest
  " 2" : RelationalOperator  Operator=>  OutDataTypeStr=boolean  RndMeth=Nearest
  " 3" : RelationalOperator  Operator=<  OutDataTypeStr=boolean  RndMeth=Nearest
  Abs : Abs
  Add : Sum
  Add1 : Sum
  Constant1 : Constant  Value=limit_selectlow
  Constant2 : Constant  Value=SH_SL_switch
  Constant3 : Constant  Value=SH_SL_switch
  Data Type Conversion : DataTypeConversion
  Data Type Conversion1 : DataTypeConversion
  Data Type Conversion2 : DataTypeConversion
  Logical Operator : Logic  AllPortsSameDT=off  OutDataTypeStr=boolean
  Logical Operator1 : Logic  Operator=OR  AllPortsSameDT=off  OutDataTypeStr=boolean
  Subtract : Sum  Inputs=+-
  Subtract1 : Sum  Inputs=+-
  Subtract2 : Sum  Inputs=+-
  vquer_HA : Gain  Gain=0.5
  vquer_HA2 : Gain  Gain=10
  vquer_HA3 : Gain  Gain=20
  category : Outport  VectorParamsAs1DForOutWhenUnconnected=off
  wires:
  v_undrivenR/1 -> Add/2, Subtract1/2
  Add/1 -> vquer_HA/1
  v_undrivenL/1 -> Add/1, Subtract/2
  vquer_HA/1 -> " 2"/1, " 1"/1
  vquer_HA2/1 -> Add1/1
  vquer_HA3/1 -> Add1/2
  Add1/1 -> Data Type Conversion/1
  Data Type Conversion/1 -> category/1
  Logical Operator1/1 -> Data Type Conversion2/1
  " 1"/1 -> Logical Operator/2
  Logical Operator/1 -> Data Type Conversion1/1
  v_drivenL/1 -> Subtract/1
  v_drivenR/1 -> Subtract1/1
  Subtract1/1 -> Subtract2/1
  Subtract/1 -> Subtract2/2
  Subtract2/1 -> Abs/1
  " "/1 -> Logical Operator/1
  " 3"/1 -> Logical Operator1/2
  Abs/1 -> " 3"/1, " "/1
  Constant2/1 -> " "/2
  Constant1/1 -> " 2"/2, " 1"/2
  " 2"/1 -> Logical Operator1/1
  Constant3/1 -> " 3"/2
  Data Type Conversion1/1 -> vquer_HA2/1
  Data Type Conversion2/1 -> vquer_HA3/1

== system HydBrakeCU_ESP/CarMaker/IPG Vehicle/Brake/HydBrakeCU Example/ESP Controller/ESP General System/ASR/MSR ECU/MSR logic/operating mode ==
  note: Criteria of modes (Arbeitsbereiche) - Burckhardt: Fahrwerktechnik p.174f.
  v_undrivenL : Inport
  v_undrivenR : Inport  Port=2
  " " : RelationalOperator  OutDataTypeStr=boolean  RndMeth=Nearest
  " 1" : RelationalOperator  Operator=<=  OutDataTypeStr=boolean  RndMeth=Nearest
  " 2" : RelationalOperator  Operator=>  OutDataTypeStr=boolean  RndMeth=Nearest
  " 3" : RelationalOperator  Operator=<=  OutDataTypeStr=boolean  RndMeth=Nearest
  AB1 = inaktiv : simulink/Logic and Bit Operations/Compare To Constant  relop=<  const=1  OutDataTypeStr=uint8
  AB1 = inaktiv1 : simulink/Logic and Bit Operations/Compare To Constant  relop=<  const=1  OutDataTypeStr=uint8
  Abs : Abs
  Add : Sum
  Add1 : Sum  Inputs=+++
  Constant1 : Constant  Value=limit_starting
  Constant2 : Constant  Value=limit_acc
  Constant3 : Constant  Value=limit_vdiff
  Constant4 : Constant  Value=MPS2KMPH
  Data Type Conversion{,1..3} (4 alike) : DataTypeConversion
  Derivative : Derivative
  Discrete Filter : DiscreteFilter  Numerator=wheelspeed_filter_num  Denominator=wheelspeed_filter_denom  SampleTime=0.001
  Divide : Product  Inputs=*/
  Logical Operator : Logic  Inputs=3  AllPortsSameDT=off  OutDataTypeStr=boolean
  Logical Operator1 : Logic  AllPortsSameDT=off  OutDataTypeStr=boolean
  Subtract : Sum  Inputs=+-
  v_average_Rear : Gain  Gain=0.5
  vquer_HA2 : Gain
  vquer_HA3 : Gain  Gain=2
  vquer_HA4 : Gain  Gain=3
  mode : Outport  VectorParamsAs1DForOutWhenUnconnected=off
  wires:
  " 1"/1 -> AB1 = inaktiv/1, Data Type Conversion1/1  "mode1 =  active"
  Add/1 -> v_average_Rear/1
  v_undrivenL/1 -> Subtract/1, Add/1
  v_undrivenR/1 -> Add/2, Subtract/2
  v_average_Rear/1 -> " 1"/1, Divide/1, " 2"/1
  Divide/1 -> Discrete Filter/1
  Derivative/1 -> " "/1
  Subtract/1 -> Abs/1
  Abs/1 -> " 3"/1
  Logical Operator/1 -> AB1 = inaktiv1/1, Data Type Conversion2/1
  Logical Operator1/1 -> Data Type Conversion3/1
  AB1 = inaktiv/1 -> Logical Operator1/1
  AB1 = inaktiv1/1 -> Logical Operator1/2
  vquer_HA3/1 -> Add1/2  "mode = 2"
  vquer_HA4/1 -> Add1/3  "mode =3"
  vquer_HA2/1 -> Add1/1  "mode = 1"
  Add1/1 -> Data Type Conversion/1
  " 2"/1 -> Logical Operator/1
  " "/1 -> Logical Operator/2
  Data Type Conversion/1 -> mode/1
  " 3"/1 -> Logical Operator/3
  Discrete Filter/1 -> Derivative/1
  Constant1/1 -> " 2"/2, " 1"/2
  Constant2/1 -> " "/2
  Constant3/1 -> " 3"/2
  Constant4/1 -> Divide/2
  Data Type Conversion1/1 -> vquer_HA2/1
  Data Type Conversion2/1 -> vquer_HA3/1
  Data Type Conversion3/1 -> vquer_HA4/1

== system HydBrakeCU_ESP/CarMaker/IPG Vehicle/Brake/HydBrakeCU Example/ESP Controller/ESP General System/ASR/MSR ECU/MSR/Gas Controller/Enabled Subsystem ==
  In1 : Inport
  Trigger : TriggerPort  VariantControl=Variant
  Out1 : Outport  VectorParamsAs1DForOutWhenUnconnected=off
  wires:
  In1/1 -> Out1/1

== system HydBrakeCU_ESP/CarMaker/IPG Vehicle/Brake/HydBrakeCU Example/ESP Controller/ESP General System/ASR/MSR ECU/MSR/Gas Controller/PID Controller ==
  u : Inport
  RESET : Inport  Port=2
  Derivative Gain : Gain  Gain=MSR_ctrl_kD
  Filter : Integrator  ExternalReset=either
  Filter Coefficient : Gain
  Integral Gain : Gain  Gain=MSR_ctrl_kI
  Integrator : Integrator  ExternalReset=either
  Proportional Gain : Gain  Gain=MSR_ctrl_kP
  Sum : Sum  Inputs=+++
  SumD : Sum  Inputs=|+-
  y : Outport  InitialOutput=0  VectorParamsAs1DForOutWhenUnconnected=off
  wires:
  Filter/1 -> SumD/2
  RESET/1 -> Integrator/2, Filter/2
  Sum/1 -> y/1
  Integrator/1 -> Sum/2
  Filter Coefficient/1 -> Filter/1, Sum/3
  Proportional Gain/1 -> Sum/1
  Derivative Gain/1 -> SumD/1
  u/1 -> Integral Gain/1, Derivative Gain/1, Proportional Gain/1
  SumD/1 -> Filter Coefficient/1
  Integral Gain/1 -> Integrator/1

== system HydBrakeCU_ESP/CarMaker/IPG Vehicle/Brake/HydBrakeCU Example/ESP Controller/ESP General System/ESP/ECU/ECU logic/P Slip angle ==
  x : Inport
  " " : Constant  Value=PID_kP_sideslip
  epsilon11 : Product
  y : Outport  VectorParamsAs1DForOutWhenUnconnected=off
  wires:
  " "/1 -> epsilon11/1
  x/1 -> epsilon11/2
  epsilon11/1 -> y/1

== system HydBrakeCU_ESP/CarMaker/IPG Vehicle/Brake/HydBrakeCU Example/ESP Controller/ESP General System/ESP/ECU/ECU logic/P Yaw Rate ==
  x : Inport
  " " : Constant  Value=PID_kP_yawrate
  epsilon11 : Product
  y1 : Outport  VectorParamsAs1DForOutWhenUnconnected=off
  wires:
  " "/1 -> epsilon11/1
  x/1 -> epsilon11/2
  epsilon11/1 -> y1/1

== system HydBrakeCU_ESP/CarMaker/IPG Vehicle/Brake/HydBrakeCU Example/ESP Controller/ESP General System/ESP/ECU/ECU logic/Threshold correction coefficient  as regards vehicle's velocity ==
  v : Inport
  Saturation : Saturate  UpperLimit=1  LowerLimit=0
  Sum2 : Sum  Inputs=+-  InputSameDT=on  SaturateOnIntegerOverflow=on  OutDataTypeStr=Inherit: Same as first input
  b1 : Constant  Value=vel_char_lim_low
  b2 : Constant  Value=vel_char_lim_high
  b3 : Constant  Value=MPS2KMPH
  b4 : Constant  Value=MPS2KMPH
  epsilon1 : Product  Inputs=*/
  epsilon10 : Product  Inputs=/*
  epsilon2 : Product  Inputs=*/
  Threshold correction coefficient : Outport  VectorParamsAs1DForOutWhenUnconnected=off
  wires:
  epsilon10/1 -> Saturation/1
  Sum2/1 -> epsilon10/2
  v/1 -> Sum2/1
  Saturation/1 -> Threshold correction coefficient/1
  epsilon2/1 -> epsilon10/1
  b2/1 -> epsilon2/1
  b3/1 -> epsilon2/2
  b4/1 -> epsilon1/2
  b1/1 -> epsilon1/1
  epsilon1/1 -> Sum2/2

== system HydBrakeCU_ESP/CarMaker/IPG Vehicle/Brake/HydBrakeCU Example/ESP Controller/ESP General System/ESP/ECU/ECU logic/shut down ESP if v<v lim ==
  note: Transfer Fcn:
      | It enables the ESC to shut down smoothly
      | when the vehicle's velocity becomes lower than v lim
  v : Inport
  v lim ESP : Inport  Port=2
  Data Type Conversion1 : DataTypeConversion
  Gain2 : Gain  OutDataTypeStr=Inherit: Same as input
  Relational Operator : RelationalOperator  OutDataTypeStr=boolean  RndMeth=Nearest
  Transfer Fcn : TransferFcn  Denominator=[0.1 1]
  ON/OFF velocity condition : Outport  VectorParamsAs1DForOutWhenUnconnected=off
  wires:
  v/1 -> Relational Operator/1
  Transfer Fcn/1 -> ON/OFF velocity condition/1
  Relational Operator/1 -> Gain2/1
  v lim ESP/1 -> Relational Operator/2
  Gain2/1 -> Data Type Conversion1/1
  Data Type Conversion1/1 -> Transfer Fcn/1

== system HydBrakeCU_ESP/CarMaker/IPG Vehicle/Brake/HydBrakeCU Example/ESP Controller/ESP General System/ESP/ECU/Instability detectors/avoids 0 ==
  note: This value has to be low enought
      | to enable the turning radius "r" to
      | be sufficiently large, in order to avoid
      | problems when the steer angle is close to zero
      | (and that the turning radius should be infinty)
  In1 : Inport
  Compare To Zero : simulink/Logic and Bit Operations/Compare To Zero  relop=~=  OutDataTypeStr=uint8
  Constant : Constant  Value=0.00001
  Dead Zone : DeadZone  LowerValue=-0.00001  UpperValue=0.00001  SaturateOnIntegerOverflow=on
  ON/OFF : Relay  OnSwitchValue=0  OffSwitchValue=0  OffOutputValue=-1  ZeroCross=off
  Product7 : Product  RndMeth=Zero
  Switch : Switch  Criteria=u2 > Threshold
  Out1 : Outport  VectorParamsAs1DForOutWhenUnconnected=off
  wires:
  Compare To Zero/1 -> Switch/2
  Dead Zone/1 -> Compare To Zero/1, Switch/1
  Switch/1 -> Out1/1
  In1/1 -> Dead Zone/1, ON/OFF/1
  Product7/1 -> Switch/3
  Constant/1 -> Product7/2
  ON/OFF/1 -> Product7/1

== system HydBrakeCU_ESP/CarMaker/IPG Vehicle/Brake/HydBrakeCU Example/ESP Controller/ESP General System/ESP/ECU/Instability detectors/avoids 0 again ==
  note: This value has to be lower than "v lim"
      | which is used in the block "response model"
      | to desable the ESP
  In1 : Inport
  Relational Operator : RelationalOperator  OutDataTypeStr=boolean  RndMeth=Nearest
  Switch : Switch  Criteria=u2 > Threshold
  velocity (in m/s) : Constant  Value=3/3.6
  Out1 : Outport  VectorParamsAs1DForOutWhenUnconnected=off
  wires:
  Relational Operator/1 -> Switch/2
  In1/1 -> Relational Operator/1, Switch/1
  velocity (in m/s)/1 -> Relational Operator/2, Switch/3
  Switch/1 -> Out1/1

== system HydBrakeCU_ESP/CarMaker/IPG Vehicle/Brake/HydBrakeCU Example/ESP Controller/ESP General System/ESP/ECU/Motor management strategy/PID-Controller ==
  u : Inport
  RESET : Inport  Port=2
  Derivative Gain : Gain  Gain=ESP_ctrl_kD
  Filter : Integrator  ExternalReset=either
  Filter Coefficient : Gain
  Integral Gain : Gain  Gain=ESP_ctrl_kI
  Integrator : Integrator  ExternalReset=either
  Proportional Gain : Gain  Gain=ESP_ctrl_kP
  Sum : Sum  Inputs=+++
  SumD : Sum  Inputs=|+-
  y : Outport  InitialOutput=0  VectorParamsAs1DForOutWhenUnconnected=off
  wires:
  Sum/1 -> y/1
  RESET/1 -> Integrator/2, Filter/2
  Derivative Gain/1 -> SumD/1
  Integrator/1 -> Sum/2
  Filter Coefficient/1 -> Filter/1, Sum/3
  Filter/1 -> SumD/2
  Integral Gain/1 -> Integrator/1
  SumD/1 -> Filter Coefficient/1
  Proportional Gain/1 -> Sum/1
  u/1 -> Integral Gain/1, Derivative Gain/1, Proportional Gain/1

== system HydBrakeCU_ESP/CarMaker/IPG Vehicle/Brake/HydBrakeCU Example/ESP Controller/ESP General System/ESP/ECU/Motor management strategy/restoration to driver ==
  controller in : Inport
  activation on : Inport  Port=2
  driver in : Inport  Port=3
  I-Controller : Subsystem
  Saturation Dynamic1 : simulink/Discontinuities/Saturation Dynamic  OutMin=[]  OutMax=[]  OutDataTypeStr=Inherit: Same as second input  OutDataType=sfix(16)  OutScaling=2^-10  DoSatur=off
  Subtract1 : Sum  Inputs=+-
  lock_signal for n s : Subsystem
  vquer_VA4 : Gain  Gain=0
  vquer_VA5 : Gain
  Control Gas : Outport  VectorParamsAs1DForOutWhenUnconnected=off
  restoration : Outport  Port=2  VectorParamsAs1DForOutWhenUnconnected=off
  wires:
  lock_signal for n s/1(Start_value_locked) -> I-Controller/2(RESET), restoration/1
  Subtract1/1 -> I-Controller/1(u)
  I-Controller/1(y) -> Saturation Dynamic1/2
  vquer_VA4/1 -> Saturation Dynamic1/3
  vquer_VA5/1 -> Saturation Dynamic1/1
  controller in/1 -> I-Controller/3(I0), Subtract1/2
  driver in/1 -> vquer_VA4/1, vquer_VA5/1, Subtract1/1
  activation on/1 -> lock_signal for n s/1(Start_value)
  Saturation Dynamic1/1 -> Control Gas/1

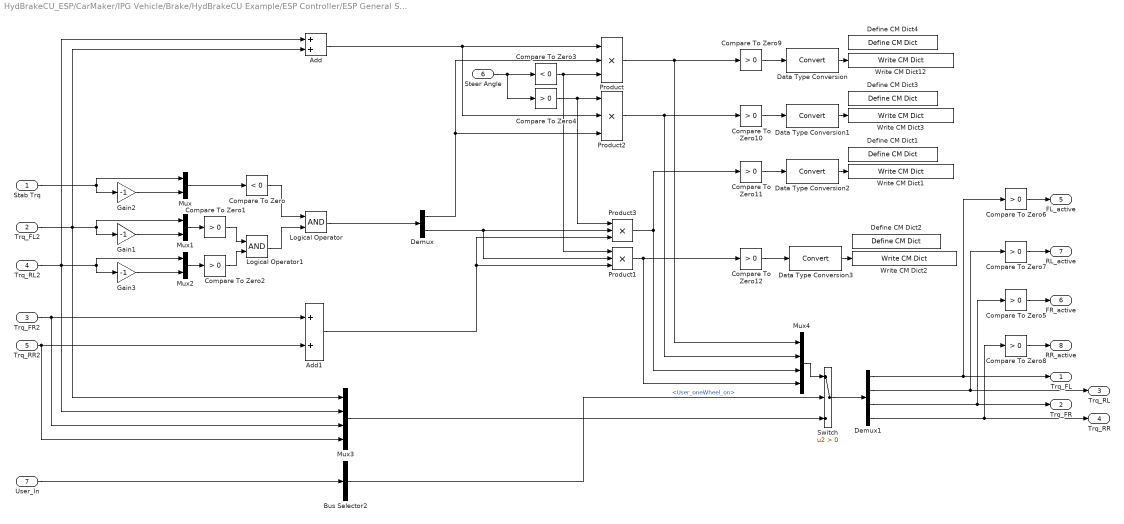
== system HydBrakeCU_ESP/CarMaker/IPG Vehicle/Brake/HydBrakeCU Example/ESP Controller/ESP General System/ESP/ECU/brake distribution strategy/2Rad ->1Rad ==
  Stab Trq : Inport
  Trq_FL2 : Inport  Port=2
  Trq_FR2 : Inport  Port=3
  Trq_RL2 : Inport  Port=4
  Trq_RR2 : Inport  Port=5
  Steer Angle : Inport  Port=6
  User_In : Inport  Port=7
  Add : Sum
  Add1 : Sum
  Bus Selector2 : BusSelector  OutputSignals=User_oneWheel_on
  Compare To Zero : simulink/Logic and Bit Operations/Compare To Zero  relop=<  OutDataTypeStr=uint8
  Compare To Zero{1..2,4..12} (11 alike) : simulink/Logic and Bit Operations/Compare To Zero  relop=>  OutDataTypeStr=uint8
  Compare To Zero3 : simulink/Logic and Bit Operations/Compare To Zero  relop=<  OutDataTypeStr=uint8
  Data Type Conversion{,1..3} (4 alike) : DataTypeConversion
  Define CM Dict1 : CarMaker4SL/Define CM Dict  xname=ESP.FR_active  xmono=off  xtype=Char  xdvaplace=VC  xnstates=2  xfirststate=0  xinitial=0
  Define CM Dict2 : CarMaker4SL/Define CM Dict  xname=ESP.RR_active  xmono=off  xtype=Char  xdvaplace=VC  xnstates=2  xfirststate=0  xinitial=0
  Define CM Dict3 : CarMaker4SL/Define CM Dict  xname=ESP.RL_active  xmono=off  xtype=Char  xdvaplace=VC  xnstates=2  xfirststate=0  xinitial=0
  Define CM Dict4 : CarMaker4SL/Define CM Dict  xname=ESP.FL_active  xmono=off  xtype=Char  xdvaplace=VC  xnstates=2  xfirststate=0  xinitial=0
  Demux : Demux  Outputs=2
  Demux1 : Demux
  Gain1 : Gain  Gain=-1
  Gain2 : Gain  Gain=-1
  Gain3 : Gain  Gain=-1
  Logical Operator : Logic  AllPortsSameDT=off
  Logical Operator1 : Logic  AllPortsSameDT=off  OutDataTypeStr=boolean
  Mux : Mux  Inputs=2
  Mux1 : Mux  Inputs=2
  Mux2 : Mux  Inputs=2
  Mux3 : Mux
  Mux4 : Mux
  Product{,1..3} (4 alike) : Product  Inputs=3  RndMeth=Zero
  Switch : Switch  Criteria=u2 > Threshold
  Write CM Dict1 : CarMaker4SL/Write CM Dict  xname=ESP.FR_active  xsync=off
  Write CM Dict12 : CarMaker4SL/Write CM Dict  xname=ESP.FL_active  xsync=off
  Write CM Dict2 : CarMaker4SL/Write CM Dict  xname=ESP.RR_active  xsync=off
  Write CM Dict3 : CarMaker4SL/Write CM Dict  xname=ESP.RL_active  xsync=off
  Trq_FL : Outport  VectorParamsAs1DForOutWhenUnconnected=off
  Trq_FR : Outport  Port=2  VectorParamsAs1DForOutWhenUnconnected=off
  Trq_RL : Outport  Port=3  VectorParamsAs1DForOutWhenUnconnected=off
  Trq_RR : Outport  Port=4  VectorParamsAs1DForOutWhenUnconnected=off
  FL_active : Outport  Port=5  VectorParamsAs1DForOutWhenUnconnected=off
  FR_active : Outport  Port=6  VectorParamsAs1DForOutWhenUnconnected=off
  RL_active : Outport  Port=7  VectorParamsAs1DForOutWhenUnconnected=off
  RR_active : Outport  Port=8  VectorParamsAs1DForOutWhenUnconnected=off
  wires:
  Compare To Zero/1 -> Logical Operator/1
  Logical Operator1/1 -> Logical Operator/2
  Logical Operator/1 -> Demux/1
  Compare To Zero1/1 -> Logical Operator1/1
  Compare To Zero2/1 -> Logical Operator1/2
  Stab Trq/1 -> Gain2/1, Mux/1
  Gain2/1 -> Mux/2
  Mux/1 -> Compare To Zero/1
  Trq_FL2/1 -> Gain1/1, Mux1/1, Add/2, Mux3/1
  Gain1/1 -> Mux1/2
  Trq_RL2/1 -> Gain3/1, Mux2/1, Add/1, Mux3/2
  Gain3/1 -> Mux2/2
  Mux2/1 -> Compare To Zero2/1
  Mux1/1 -> Compare To Zero1/1
  Add/1 -> Product/1, Product2/2
  Demux/1 -> Product/2, Product2/3
  Product/1 -> Mux4/1, Compare To Zero9/1
  Add1/1 -> Product3/3, Product1/3
  Demux/2 -> Product3/2, Product1/2
  Product3/1 -> Mux4/3, Compare To Zero11/1
  Trq_FR2/1 -> Add1/1, Mux3/3
  Trq_RR2/1 -> Add1/2, Mux3/4
  Steer Angle/1 -> Compare To Zero3/1, Compare To Zero4/1
  Compare To Zero3/1 -> Product/3, Product1/1
  Product2/1 -> Mux4/2, Compare To Zero10/1
  Compare To Zero4/1 -> Product2/1, Product3/1
  Product1/1 -> Mux4/4, Compare To Zero12/1
  Compare To Zero6/1 -> FL_active/1
  Compare To Zero7/1 -> RL_active/1
  Compare To Zero8/1 -> RR_active/1
  Data Type Conversion/1 -> Write CM Dict12/1
  Mux3/1 -> Switch/3
  Mux4/1 -> Switch/1
  Switch/1 -> Demux1/1
  Demux1/1 -> Trq_FL/1, Compare To Zero6/1
  Demux1/2 -> Trq_RL/1, Compare To Zero7/1
  Demux1/3 -> Trq_FR/1, Compare To Zero5/1
  Demux1/4 -> Trq_RR/1, Compare To Zero8/1
  Bus Selector2/1 -> Switch/2  "<User_oneWheel_on>"
  Compare To Zero9/1 -> Data Type Conversion/1
  Data Type Conversion1/1 -> Write CM Dict3/1
  Compare To Zero10/1 -> Data Type Conversion1/1
  Compare To Zero11/1 -> Data Type Conversion2/1
  Data Type Conversion2/1 -> Write CM Dict1/1
  Data Type Conversion3/1 -> Write CM Dict2/1
  Compare To Zero5/1 -> FR_active/1
  Compare To Zero12/1 -> Data Type Conversion3/1
  User_In/1 -> Bus Selector2/1
